simulink model "Ignorant"  (R2023b)
settings: Solver=VariableStepAuto  StartTime=0.0  StopTime=9  RelTol=1e-3
model workspace: external: MATLAB File D:\College\Senior 2\GP\Delta\Design\INSHALLAAHHHHH\SSCPE\25Mar\Ignorant_DataFile.m (data not in the file)
values from neighbouring files (symbols this model uses):
  X = [0 -180 -180 -180 180 180 180 180 0]    [Simulaiton_Main.m]    (also in csp_XYZ.m; csp_XYZ_X.m = [-180 -180]; csp_XYZ_circular_motion.m = center(1) + radius * cos(theta); csp_angles.m)
  Y = zeros(1,numel(X_3ars))    [CSPPPPPPPPPPPPpp.m]    (also in Simulaiton_Main.m = zeros(1,9); csp_XYZ.m = zeros(1,9); csp_XYZ_X.m = [0 0]; csp_XYZ_circular_motion.m = center(2) + radius * sin(theta))
  Z = -400*ones(1,numel(X_3ars))    [CSPPPPPPPPPPPPpp.m]    (also in Simulaiton_Main.m = [-300 -300 -400 -300 -300 -300 -400 -300 -300]; csp_XYZ.m = [-300 -300 -400 -300 -300 -300 -400 -300 -300]; csp_XYZ_X.m = [-300 -500]; csp_XYZ_circular_motion.m = center(3) * ones(size(X)))
undefined symbols (not defined in the file or in its folder): smiData
libraries: sm_lib x390, nesl_utility x4
(part 1 of 8)
settings Model: Creator=Dell  LastModifiedBy=Dell

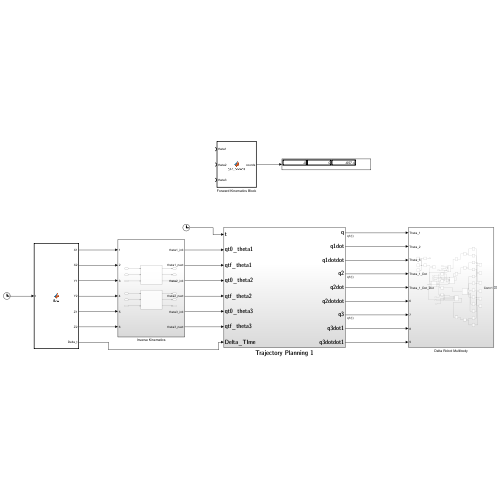
[thumbnail: Simulink's stored preview of the top-level diagram]
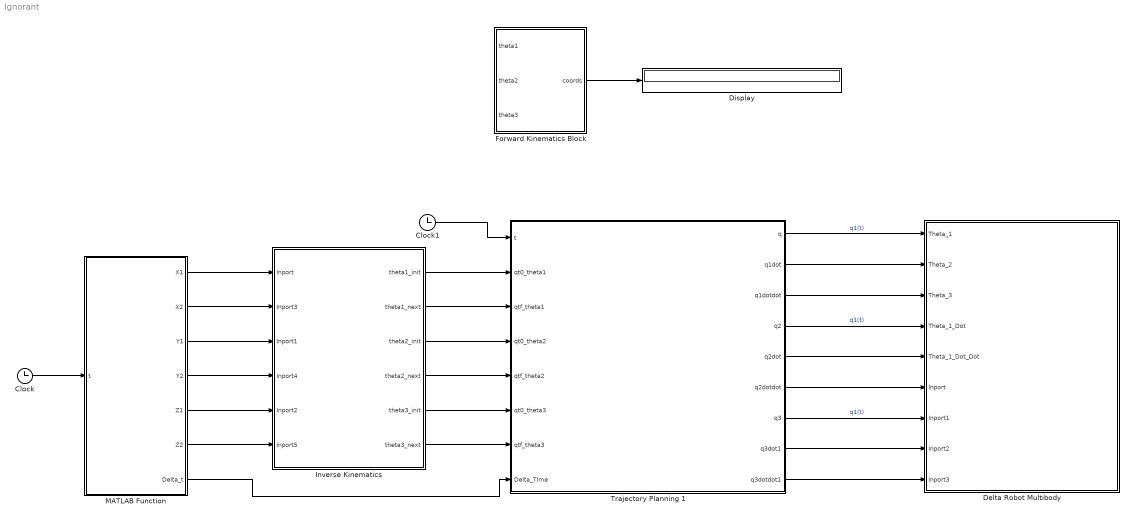
== system Ignorant ==
  Clock : Clock
  Clock1 : Clock
  Delta Robot Multibody : Subsystem
  Display : Display
  Forward Kinematics Block : MATLAB Function  TreatAsAtomicUnit=on
  Inverse Kinematics : Subsystem
  MATLAB Function : MATLAB Function  TreatAsAtomicUnit=on
  Trajectory Planning 1 : Subsystem
  wires:
  Forward Kinematics Block/1(coords) -> Display/1
  Clock/1 -> MATLAB Function/1(t)
  Inverse Kinematics/1(theta1_init) -> Trajectory Planning 1/2(qt0_theta1)
  Trajectory Planning 1/1(q) -> Delta Robot Multibody/1(Theta_1)  "q1(t)"
  Trajectory Planning 1/2(q1dot) -> Delta Robot Multibody/2(Theta_2)
  Trajectory Planning 1/3(q1dotdot) -> Delta Robot Multibody/3(Theta_3)
  Trajectory Planning 1/4(q2) -> Delta Robot Multibody/4(Theta_1_Dot)  "q1(t)"
  Trajectory Planning 1/5(q2dot) -> Delta Robot Multibody/5(Theta_1_Dot_Dot)
  Trajectory Planning 1/6(q2dotdot) -> Delta Robot Multibody/6(Inport)
  Trajectory Planning 1/7(q3) -> Delta Robot Multibody/7(Inport1)  "q1(t)"
  Trajectory Planning 1/8(q3dot1) -> Delta Robot Multibody/8(Inport2)
  Trajectory Planning 1/9(q3dotdot1) -> Delta Robot Multibody/9(Inport3)
  Clock1/1 -> Trajectory Planning 1/1(t)
  MATLAB Function/1(X1) -> Inverse Kinematics/1(Inport)
  MATLAB Function/6(Z2) -> Inverse Kinematics/6(Inport5)
  MATLAB Function/7(Delta_t) -> Trajectory Planning 1/8(Delta_TIme)
  MATLAB Function/5(Z1) -> Inverse Kinematics/5(Inport2)
  MATLAB Function/3(Y1) -> Inverse Kinematics/3(Inport1)
  MATLAB Function/2(X2) -> Inverse Kinematics/2(Inport3)
  MATLAB Function/4(Y2) -> Inverse Kinematics/4(Inport4)
  Inverse Kinematics/2(theta1_next) -> Trajectory Planning 1/3(qtf_theta1)
  Inverse Kinematics/3(theta2_init) -> Trajectory Planning 1/4(qt0_theta2)
  Inverse Kinematics/4(theta2_next) -> Trajectory Planning 1/5(qtf_theta2)
  Inverse Kinematics/5(theta3_init) -> Trajectory Planning 1/6(qt0_theta3)
  Inverse Kinematics/6(theta3_next) -> Trajectory Planning 1/7(qtf_theta3)
